simulink model "kinctrlkinova"  (Simulink 10.3)
settings: Solver=ode45  StartTime=0.0  StopTime=30  MaxStep=0.1  RelTol=1e-5  EnableMultiTasking=on
values from neighbouring files (symbols this model uses):
  ff = ctrl    [eval_mod.m]    (also in sim_q1.m = i)
  k = [1 1;1 1;1 1]    [eval_mod.m]    (also in sim_q3.m = 1)
  n = i    [eval_mod.m]    (also in sim_q1.m = j)
  q0 = [0, 15, 180, -130, 0, 55, 90]    [mdl_kinovagen3_trab2.m]    (also in mdl_planar_2r.m = [-pi/20, -pi/2])
libraries: roblocks x4, simulink x1
settings Model: Creator=fernando  LastModifiedBy=Guga
settings DataIOCC: LimitDataPoints=on  ReturnWorkspaceOutputs=on
settings DebuggingCC: SolverPrmCheckMsg=warning  AllowSymbolicDim=off

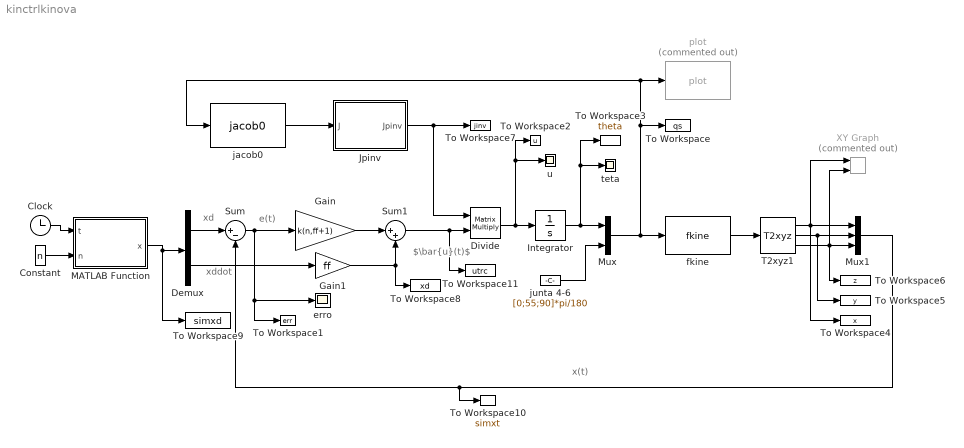
== system kinctrlkinova ==
  note: x(t)
  note: xd
  note: xddot
  note: e(t)
  note: $\bar{u}(t)$
  Clock : Clock
  Constant : Constant  Value=n
  Demux : Demux  Outputs=2
  Divide : Product  Inputs=**  Multiplication=Matrix(*)
  Gain : Gain  Gain=k(n,ff+1)
  Gain1 : Gain  Gain=ff
  Integrator : Integrator  InitialCondition=q0(1:4)*pi/180
  Jpinv : MATLAB Function  TreatAsAtomicUnit=on
  MATLAB Function : MATLAB Function  TreatAsAtomicUnit=on
  Mux : Mux  Inputs=2
  Mux1 : Mux  Inputs=3
  Sum : Sum  Inputs=|+-
  Sum1 : Sum  Inputs=|++
  T2xyz1 : roblocks/Toolbox/T2xyz
  To Workspace : ToWorkspace  VariableName=qs  SaveFormat=Timeseries  SampleTime=-1
  To Workspace1 : ToWorkspace  VariableName=err  SaveFormat=Timeseries  SampleTime=-1
  To Workspace10 : ToWorkspace  VariableName=simxt  SaveFormat=Timeseries  SampleTime=-1
  To Workspace11 : ToWorkspace  VariableName=utrc  SaveFormat=Timeseries  SampleTime=-1
  To Workspace2 : ToWorkspace  VariableName=u  SaveFormat=Timeseries  SampleTime=-1
  To Workspace3 : ToWorkspace  VariableName=theta  SaveFormat=Timeseries  SampleTime=-1
  To Workspace4 : ToWorkspace  VariableName=x  SaveFormat=Timeseries  SampleTime=-1
  To Workspace5 : ToWorkspace  VariableName=y  SaveFormat=Timeseries  SampleTime=-1
  To Workspace6 : ToWorkspace  VariableName=z  SaveFormat=Timeseries  SampleTime=-1
  To Workspace7 : ToWorkspace  VariableName=jinv  SaveFormat=Timeseries  SampleTime=-1
  To Workspace8 : ToWorkspace  VariableName=xd  SaveFormat=Timeseries  SampleTime=-1
  To Workspace9 : ToWorkspace  VariableName=simxd  SaveFormat=Timeseries  SampleTime=-1
  XY Graph : simulink/Sinks/XY Graph  Commented=on  xmin=-1  xmax=1  ymin=-1  ymax=1  st=-1
  erro : Scope
  fkine : roblocks/Arm/fkine  robot=gen3
  "jacob0 " : roblocks/Arm/jacob0   robot=gen3
  junta 4-6 : Constant  Value=[0;55;90]*pi/180
  plot : roblocks/Arm/plot  Commented=on  robot=gen3  fps=5  holdplot=on
  teta : Scope
  u : Scope
  wires:
  Integrator/1 -> Mux/1, To Workspace3/1, teta/1
  junta 4-6/1 -> Mux/2
  Divide/1 -> Integrator/1, u/1, To Workspace2/1
  Jpinv/1(Jpinv) -> To Workspace7/1, Divide/1
  Sum/1 -> Gain/1, erro/1, To Workspace1/1
  fkine/1 -> T2xyz1/1
  T2xyz1/1 -> XY Graph/1, Mux1/1, To Workspace4/1
  T2xyz1/2 -> To Workspace5/1, Mux1/2
  T2xyz1/3 -> To Workspace6/1, Mux1/3, XY Graph/2
  Mux1/1 -> To Workspace10/1, Sum/2
  "jacob0 "/1 -> Jpinv/1(J)
  Clock/1 -> MATLAB Function/1(t)
  MATLAB Function/1(x) -> To Workspace9/1, Demux/1
  Demux/1 -> Sum/1
  Gain/1 -> Sum1/1
  Demux/2 -> Gain1/1
  Sum1/1 -> To Workspace11/1, Divide/2
  Constant/1 -> MATLAB Function/2(n)
  Mux/1 -> fkine/1, To Workspace/1, "jacob0 "/1, plot/1
  Gain1/1 -> Sum1/2, To Workspace8/1

== matlab function Jpinv ==
  data: J input double; Jpinv output double
function Jpinv = fcn(J)
%#codegen

Jpinv = pinv(J(1:3,1:4));

== matlab function MATLAB Function ==
  data: t input double; x output double; n input double
function x = trajectories(t,n)
wn = 2*pi/10;   
    switch n
        case 1
            x = [0.1*cos(wn*t) + 0.4; 0 ;0.1*sin(wn*t) + 0.4;-wn*0.1*sin(wn*t);0 ; wn*0.1*cos(wn*t) ];
        case 2
            x = [0.1*cos(wn*t)+0.4;0.1*cos(wn*t)+0.1*sin(wn*t);0.1*sin(wn*t)+0.4;-wn*0.1*sin(wn*t);
                -wn*0.1*sin(wn*t)+wn*0.1*cos(wn*t);wn*0.1*cos(wn*t)];
        case 3
            x = [0.08*(sin(wn*t)+sin(4*wn*t))+ 0.4;0;0.08*(cos(wn*t)+cos(4*wn*t))+ 0.4;
                0.08*(wn*cos(wn*t)+4*wn*cos(4*wn*t));0;0.08*(-wn*sin(wn*t)-4*wn*sin(4*wn*t))];
        otherwise
            x = [0;0;0;0;0;0];
    end
end
